simulink model "Fourteen_bus"  (R2023b)
settings: Solver=ode23t  StartTime=0.0  StopTime=10  FixedStep=0.2  RelTol=1e-4  AbsTol=1e-6  EnableMultiTasking=on
undefined symbols (not defined in the file): D1, Delta
libraries: spsThreePhaseVIMeasurementLib x28, spsThreePhaseSeriesRLCBranchLib x20, spsThreePhaseSeriesRLCLoadLib x13, spsThreePhaseSourceLib x4, spsThreePhaseTransformerTwoWindingsLib x4, spsThreePhaseBreakerLib x3, spsSeriesRLCBranchLib x2, spsDCMachineLib x1, dspnetwork x1, spsUniversalBridgeLib x1, spspowerguiLib x1
(part 2 of 2)

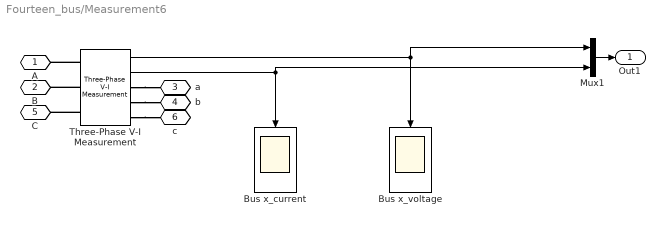
== system Fourteen_bus/Measurement6 ==
  Bus x_current : Scope
  Bus x_voltage : Scope
  Mux1 : Mux  Inputs=2
  Three-Phase V-I Measurement : spsThreePhaseVIMeasurementLib/Three-Phase V-I Measurement  VoltageMeasurement=phase-to-ground  SetLabelV=off  LabelV=Vabc  Vpu=off  VpuLL=off  CurrentMeasurement=yes  SetLabelI=off  LabelI=Iabc  Ipu=off  Pbase=100e6  Vbase=500e3  OutputType=Complex  PhasorSimulation=off  PSBequivalent=0
  A : PMIOPort  Side=Left
  B : PMIOPort  Port=2  Side=Left
  a : PMIOPort  Port=3  Side=Right
  b : PMIOPort  Port=4  Side=Right
  C : PMIOPort  Port=5  Side=Left
  c : PMIOPort  Port=6  Side=Right
  Out1 : Outport
  wires:
  Three-Phase V-I Measurement/2 -> Mux1/2, Bus x_current/1
  Three-Phase V-I Measurement/1 -> Mux1/1, Bus x_voltage/1
  Mux1/1 -> Out1/1
  connections:
  Three-Phase V-I Measurement/RConn2 -- b/RConn1
  Three-Phase V-I Measurement/LConn1 -- A/RConn1
  Three-Phase V-I Measurement/LConn2 -- B/RConn1
  Three-Phase V-I Measurement/RConn3 -- c/RConn1
  Three-Phase V-I Measurement/LConn3 -- C/RConn1
  Three-Phase V-I Measurement/RConn1 -- a/RConn1

== system Fourteen_bus/Measurement7 ==
  Bus x_current : Scope
  Bus x_voltage : Scope
  Mux1 : Mux  Inputs=2
  Three-Phase V-I Measurement : spsThreePhaseVIMeasurementLib/Three-Phase V-I Measurement  VoltageMeasurement=phase-to-ground  SetLabelV=off  LabelV=Vabc  Vpu=off  VpuLL=off  CurrentMeasurement=yes  SetLabelI=off  LabelI=Iabc  Ipu=off  Pbase=100e6  Vbase=500e3  OutputType=Complex  PhasorSimulation=off  PSBequivalent=0
  A : PMIOPort  Side=Left
  B : PMIOPort  Port=2  Side=Left
  a : PMIOPort  Port=3  Side=Right
  b : PMIOPort  Port=4  Side=Right
  C : PMIOPort  Port=5  Side=Left
  c : PMIOPort  Port=6  Side=Right
  Out1 : Outport
  wires:
  Three-Phase V-I Measurement/2 -> Mux1/2, Bus x_current/1
  Three-Phase V-I Measurement/1 -> Mux1/1, Bus x_voltage/1
  Mux1/1 -> Out1/1
  connections:
  Three-Phase V-I Measurement/RConn2 -- b/RConn1
  Three-Phase V-I Measurement/LConn1 -- A/RConn1
  Three-Phase V-I Measurement/LConn2 -- B/RConn1
  Three-Phase V-I Measurement/RConn3 -- c/RConn1
  Three-Phase V-I Measurement/LConn3 -- C/RConn1
  Three-Phase V-I Measurement/RConn1 -- a/RConn1

== system Fourteen_bus/Measurement8 ==
  Bus x_current : Scope
  Bus x_voltage : Scope
  Mux1 : Mux  Inputs=2
  Three-Phase V-I Measurement : spsThreePhaseVIMeasurementLib/Three-Phase V-I Measurement  VoltageMeasurement=phase-to-ground  SetLabelV=off  LabelV=Vabc  Vpu=off  VpuLL=off  CurrentMeasurement=yes  SetLabelI=off  LabelI=Iabc  Ipu=off  Pbase=100e6  Vbase=500e3  OutputType=Complex  PhasorSimulation=off  PSBequivalent=0
  A : PMIOPort  Side=Left
  B : PMIOPort  Port=2  Side=Left
  a : PMIOPort  Port=3  Side=Right
  b : PMIOPort  Port=4  Side=Right
  C : PMIOPort  Port=5  Side=Left
  c : PMIOPort  Port=6  Side=Right
  Out1 : Outport
  wires:
  Three-Phase V-I Measurement/2 -> Mux1/2, Bus x_current/1
  Three-Phase V-I Measurement/1 -> Mux1/1, Bus x_voltage/1
  Mux1/1 -> Out1/1
  connections:
  Three-Phase V-I Measurement/RConn2 -- b/RConn1
  Three-Phase V-I Measurement/LConn1 -- A/RConn1
  Three-Phase V-I Measurement/LConn2 -- B/RConn1
  Three-Phase V-I Measurement/RConn3 -- c/RConn1
  Three-Phase V-I Measurement/LConn3 -- C/RConn1
  Three-Phase V-I Measurement/RConn1 -- a/RConn1

== system Fourteen_bus/Measurement9 ==
  Bus x_current : Scope
  Bus x_voltage : Scope
  Mux1 : Mux  Inputs=2
  Three-Phase V-I Measurement : spsThreePhaseVIMeasurementLib/Three-Phase V-I Measurement  VoltageMeasurement=phase-to-ground  SetLabelV=off  LabelV=Vabc  Vpu=off  VpuLL=off  CurrentMeasurement=yes  SetLabelI=off  LabelI=Iabc  Ipu=off  Pbase=100e6  Vbase=500e3  OutputType=Complex  PhasorSimulation=off  PSBequivalent=0
  A : PMIOPort  Side=Left
  B : PMIOPort  Port=2  Side=Left
  a : PMIOPort  Port=3  Side=Right
  b : PMIOPort  Port=4  Side=Right
  C : PMIOPort  Port=5  Side=Left
  c : PMIOPort  Port=6  Side=Right
  Out1 : Outport
  wires:
  Three-Phase V-I Measurement/2 -> Mux1/2, Bus x_current/1
  Three-Phase V-I Measurement/1 -> Mux1/1, Bus x_voltage/1
  Mux1/1 -> Out1/1
  connections:
  Three-Phase V-I Measurement/RConn2 -- b/RConn1
  Three-Phase V-I Measurement/LConn1 -- A/RConn1
  Three-Phase V-I Measurement/LConn2 -- B/RConn1
  Three-Phase V-I Measurement/RConn3 -- c/RConn1
  Three-Phase V-I Measurement/LConn3 -- C/RConn1
  Three-Phase V-I Measurement/RConn1 -- a/RConn1

== system Fourteen_bus/UDP send ==
  In1 : Inport
  Data Type Conversion : DataTypeConversion  OutDataTypeStr=single  SaturateOnIntegerOverflow=off  RndMeth=Floor
  UDP Send : dspnetwork/UDP Send  remoteURL='127.0.0.1'  remotePort=25000  localURL='0.0.0.0'  localPortSource=Automatically determine  localPort=-1  sendBufferSize=8192  sampletime=-1  blockPlatform=[]  separateLengthPort=0
      settings: LibrarySourceBlock=dspsnks4/UDP Send
  wires:
  Data Type Conversion/1 -> UDP Send/1
  In1/1 -> Data Type Conversion/1
